simulink model "DOF2_Test2_arch"  (R2022b)
settings: Solver=VariableStepAuto  StartTime=0.0  StopTime=10.0  RelTol=1e-3
settings Model: Creator=shailesh suthar  LastModifiedBy=shailesh suthar
settings DebuggingCC: UnconnectedInputMsg=warning  UnconnectedOutputMsg=warning  UnconnectedLineMsg=warning
settings ModelReferenceCC: EnableRefExpFcnMdlSchedulingChecks=on
settings RTWCC: DLArmComputeVersion=19.05

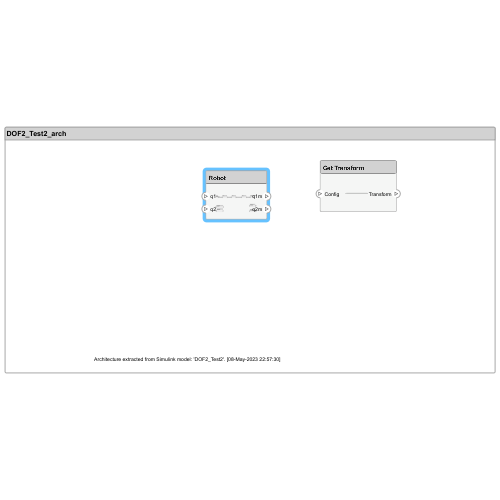
[thumbnail: Simulink's stored preview of the top-level diagram]
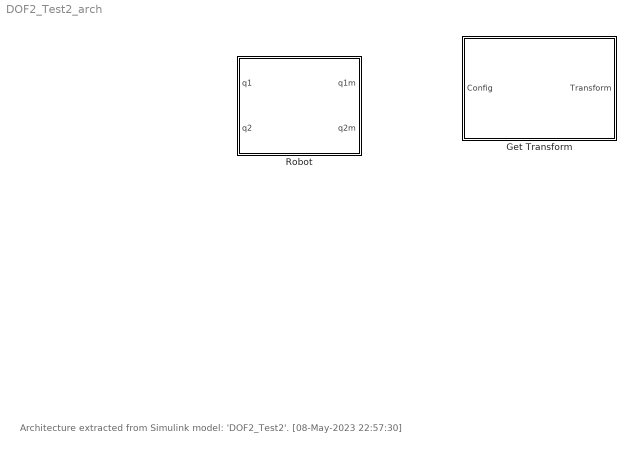
== system DOF2_Test2_arch ==
  note: Architecture extracted from Simulink model: 'DOF2_Test2'. [08-May-2023 22:57:30]
  Get Transform : Subsystem
      settings: PortSchema="{\"entries\":[{\"content\":{\"headerSize\":26,\"margin\":15,\"minimumSpacing\":25,\"sides\":[{\"content\":{\"connectorIds\":[\"In1\"]},\"type\":\"ConnectorPlacement.EquallySpacedRectSide\",\"uuid\":\"557e2789-5bde-45a7-9208-ef64bda35799\"},{\"content\":{\"connectorIds\":[\"Out1\"],\"side\":\"RIGHT\"},\"type\":\"ConnectorPlacement.EquallySpacedRectSide\",\"uuid\":\"adadcf43-a05c-4dbc-9e15-d3b2757a8feb\"},{\"content\":{\"connectorIds\":[],\"side\":\"TOP\"},\"type\":\"ConnectorPlacement.EquallySpacedRectSide\",\"uuid\":\"69984c12-afd6-46f7-91b1-af5b61a3164f\"}]},\"type\":\"ConnectorPlacement.EquallySpacedConnector\",\"uuid\":\"3da93d72-b13d-4c5c-bd73-b6426386ab06\"}],\"packageUris\":[\"http://schema.mathworks.com/mf0/Connector/R2020b\"],\"version\":\"1.0\"}"
  Robot : Subsystem
      settings: PortSchema="{\"entries\":[{\"content\":{\"headerSize\":26,\"margin\":15,\"minimumSpacing\":25,\"sides\":[{\"content\":{\"connectorIds\":[\"In1\",\"In2\"]},\"type\":\"ConnectorPlacement.EquallySpacedRectSide\",\"uuid\":\"557e2789-5bde-45a7-9208-ef64bda35799\"},{\"content\":{\"connectorIds\":[\"Out1\",\"Out2\"],\"side\":\"RIGHT\"},\"type\":\"ConnectorPlacement.EquallySpacedRectSide\",\"uuid\":\"adadcf43-a05c-4dbc-9e15-d3b2757a8feb\"},{\"content\":{\"connectorIds\":[],\"side\":\"TOP\"},\"type\":\"ConnectorPlacement.EquallySpacedRectSide\",\"uuid\":\"69984c12-afd6-46f7-91b1-af5b61a3164f\"}]},\"type\":\"ConnectorPlacement.EquallySpacedConnector\",\"uuid\":\"3da93d72-b13d-4c5c-bd73-b6426386ab06\"}],\"packageUris\":[\"http://schema.mathworks.com/mf0/Connector/R2020b\"],\"version\":\"1.0\"}"

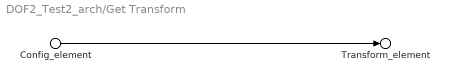
== system DOF2_Test2_arch/Get Transform ==
  Config_element : Inport  PortName=Config
  Transform_element : Outport  PortName=Transform
  wires:
  Config_element/1 -> Transform_element/1

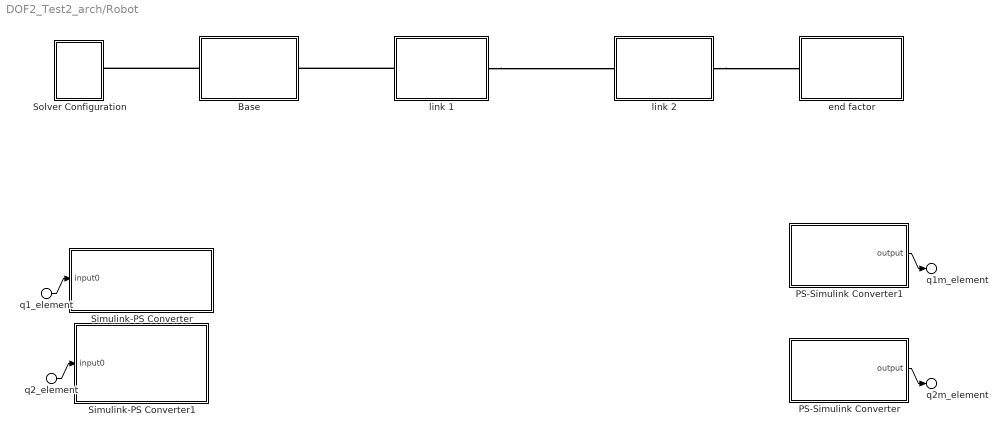
== system DOF2_Test2_arch/Robot ==
  q1_element : Inport  PortName=q1
  q2_element : Inport  Port=2  PortName=q2
  Base : Subsystem
      settings: PortSchema="{\"entries\":[{\"content\":{\"headerSize\":26,\"margin\":15,\"minimumSpacing\":25,\"sides\":[{\"content\":{\"connectorIds\":[\"LConn1\"]},\"type\":\"ConnectorPlacement.EquallySpacedRectSide\",\"uuid\":\"557e2789-5bde-45a7-9208-ef64bda35799\"},{\"content\":{\"connectorIds\":[\"RConn1\"],\"side\":\"RIGHT\"},\"type\":\"ConnectorPlacement.EquallySpacedRectSide\",\"uuid\":\"adadcf43-a05c-4dbc-9e15-d3b2757a8feb\"},{\"content\":{\"connectorIds\":[],\"side\":\"TOP\"},\"type\":\"ConnectorPlacement.EquallySpacedRectSide\",\"uuid\":\"69984c12-afd6-46f7-91b1-af5b61a3164f\"}]},\"type\":\"ConnectorPlacement.EquallySpacedConnector\",\"uuid\":\"3da93d72-b13d-4c5c-bd73-b6426386ab06\"}],\"packageUris\":[\"http://schema.mathworks.com/mf0/Connector/R2020b\"],\"version\":\"1.0\"}"
  PS-Simulink Converter : Subsystem  mask{Frequencies=[]}
      settings: PortSchema="{\"entries\":[{\"content\":{\"headerSize\":26,\"margin\":15,\"minimumSpacing\":25,\"sides\":[{\"content\":{\"connectorIds\":[\"LConn1\"]},\"type\":\"ConnectorPlacement.EquallySpacedRectSide\",\"uuid\":\"557e2789-5bde-45a7-9208-ef64bda35799\"},{\"content\":{\"connectorIds\":[\"Out1\"],\"side\":\"RIGHT\"},\"type\":\"ConnectorPlacement.EquallySpacedRectSide\",\"uuid\":\"adadcf43-a05c-4dbc-9e15-d3b2757a8feb\"},{\"content\":{\"connectorIds\":[],\"side\":\"TOP\"},\"type\":\"ConnectorPlacement.EquallySpacedRectSide\",\"uuid\":\"69984c12-afd6-46f7-91b1-af5b61a3164f\"}]},\"type\":\"ConnectorPlacement.EquallySpacedConnector\",\"uuid\":\"3da93d72-b13d-4c5c-bd73-b6426386ab06\"}],\"packageUris\":[\"http://schema.mathworks.com/mf0/Connector/R2020b\"],\"version\":\"1.0\"}"
  PS-Simulink Converter1 : Subsystem  mask{Frequencies=[]}
      settings: PortSchema="{\"entries\":[{\"content\":{\"headerSize\":26,\"margin\":15,\"minimumSpacing\":25,\"sides\":[{\"content\":{\"connectorIds\":[\"LConn1\"]},\"type\":\"ConnectorPlacement.EquallySpacedRectSide\",\"uuid\":\"557e2789-5bde-45a7-9208-ef64bda35799\"},{\"content\":{\"connectorIds\":[\"Out1\"],\"side\":\"RIGHT\"},\"type\":\"ConnectorPlacement.EquallySpacedRectSide\",\"uuid\":\"adadcf43-a05c-4dbc-9e15-d3b2757a8feb\"},{\"content\":{\"connectorIds\":[],\"side\":\"TOP\"},\"type\":\"ConnectorPlacement.EquallySpacedRectSide\",\"uuid\":\"69984c12-afd6-46f7-91b1-af5b61a3164f\"}]},\"type\":\"ConnectorPlacement.EquallySpacedConnector\",\"uuid\":\"3da93d72-b13d-4c5c-bd73-b6426386ab06\"}],\"packageUris\":[\"http://schema.mathworks.com/mf0/Connector/R2020b\"],\"version\":\"1.0\"}"
  Simulink-PS Converter : Subsystem  mask{Frequencies=[], NoiseParameters=[], InputFilterTimeConstant=[]}
      settings: PortSchema="{\"entries\":[{\"content\":{\"headerSize\":26,\"margin\":15,\"minimumSpacing\":25,\"sides\":[{\"content\":{\"connectorIds\":[\"In1\"]},\"type\":\"ConnectorPlacement.EquallySpacedRectSide\",\"uuid\":\"557e2789-5bde-45a7-9208-ef64bda35799\"},{\"content\":{\"connectorIds\":[\"RConn1\"],\"side\":\"RIGHT\"},\"type\":\"ConnectorPlacement.EquallySpacedRectSide\",\"uuid\":\"adadcf43-a05c-4dbc-9e15-d3b2757a8feb\"},{\"content\":{\"connectorIds\":[],\"side\":\"TOP\"},\"type\":\"ConnectorPlacement.EquallySpacedRectSide\",\"uuid\":\"69984c12-afd6-46f7-91b1-af5b61a3164f\"}]},\"type\":\"ConnectorPlacement.EquallySpacedConnector\",\"uuid\":\"3da93d72-b13d-4c5c-bd73-b6426386ab06\"}],\"packageUris\":[\"http://schema.mathworks.com/mf0/Connector/R2020b\"],\"version\":\"1.0\"}"
  Simulink-PS Converter1 : Subsystem  mask{Frequencies=[], NoiseParameters=[], InputFilterTimeConstant=[]}
      settings: PortSchema="{\"entries\":[{\"content\":{\"headerSize\":26,\"margin\":15,\"minimumSpacing\":25,\"sides\":[{\"content\":{\"connectorIds\":[\"In1\"]},\"type\":\"ConnectorPlacement.EquallySpacedRectSide\",\"uuid\":\"557e2789-5bde-45a7-9208-ef64bda35799\"},{\"content\":{\"connectorIds\":[\"RConn1\"],\"side\":\"RIGHT\"},\"type\":\"ConnectorPlacement.EquallySpacedRectSide\",\"uuid\":\"adadcf43-a05c-4dbc-9e15-d3b2757a8feb\"},{\"content\":{\"connectorIds\":[],\"side\":\"TOP\"},\"type\":\"ConnectorPlacement.EquallySpacedRectSide\",\"uuid\":\"69984c12-afd6-46f7-91b1-af5b61a3164f\"}]},\"type\":\"ConnectorPlacement.EquallySpacedConnector\",\"uuid\":\"3da93d72-b13d-4c5c-bd73-b6426386ab06\"}],\"packageUris\":[\"http://schema.mathworks.com/mf0/Connector/R2020b\"],\"version\":\"1.0\"}"
  Solver Configuration : Subsystem  mask{Tones=[], Harmonics=[], ResidualTolerance=[], ConsistencyAbsTol=[], ConsistencyRelTol=[], ConsistencyTolFactor=[], FunctionEvalNumThread=[], LocalSolverSampleTime=[], MaxNonlinIter=[], MaxModeIter=[], ImpulseIterations=[], LinearAlgebraNumThread=[], DelaysMemoryBudget=[], FilteringTimeConstant=[], PartitionMemoryBudget=[]}
      settings: PortSchema="{\"entries\":[{\"content\":{\"headerSize\":26,\"margin\":15,\"minimumSpacing\":25,\"sides\":[{\"content\":{\"connectorIds\":[]},\"type\":\"ConnectorPlacement.EquallySpacedRectSide\",\"uuid\":\"557e2789-5bde-45a7-9208-ef64bda35799\"},{\"content\":{\"connectorIds\":[\"RConn1\"],\"side\":\"RIGHT\"},\"type\":\"ConnectorPlacement.EquallySpacedRectSide\",\"uuid\":\"adadcf43-a05c-4dbc-9e15-d3b2757a8feb\"},{\"content\":{\"connectorIds\":[],\"side\":\"TOP\"},\"type\":\"ConnectorPlacement.EquallySpacedRectSide\",\"uuid\":\"69984c12-afd6-46f7-91b1-af5b61a3164f\"}]},\"type\":\"ConnectorPlacement.EquallySpacedConnector\",\"uuid\":\"3da93d72-b13d-4c5c-bd73-b6426386ab06\"}],\"packageUris\":[\"http://schema.mathworks.com/mf0/Connector/R2020b\"],\"version\":\"1.0\"}"
  end factor : Subsystem
      settings: PortSchema="{\"entries\":[{\"content\":{\"headerSize\":26,\"margin\":15,\"minimumSpacing\":25,\"sides\":[{\"content\":{\"connectorIds\":[\"LConn1\"]},\"type\":\"ConnectorPlacement.EquallySpacedRectSide\",\"uuid\":\"557e2789-5bde-45a7-9208-ef64bda35799\"},{\"content\":{\"connectorIds\":[],\"side\":\"RIGHT\"},\"type\":\"ConnectorPlacement.EquallySpacedRectSide\",\"uuid\":\"adadcf43-a05c-4dbc-9e15-d3b2757a8feb\"},{\"content\":{\"connectorIds\":[],\"side\":\"TOP\"},\"type\":\"ConnectorPlacement.EquallySpacedRectSide\",\"uuid\":\"69984c12-afd6-46f7-91b1-af5b61a3164f\"}]},\"type\":\"ConnectorPlacement.EquallySpacedConnector\",\"uuid\":\"3da93d72-b13d-4c5c-bd73-b6426386ab06\"}],\"packageUris\":[\"http://schema.mathworks.com/mf0/Connector/R2020b\"],\"version\":\"1.0\"}"
  link 1 : Subsystem
      settings: PortSchema="{\"entries\":[{\"content\":{\"headerSize\":26,\"margin\":15,\"minimumSpacing\":25,\"sides\":[{\"content\":{\"connectorIds\":[\"LConn1\"]},\"type\":\"ConnectorPlacement.EquallySpacedRectSide\",\"uuid\":\"557e2789-5bde-45a7-9208-ef64bda35799\"},{\"content\":{\"connectorIds\":[\"RConn1\"],\"side\":\"RIGHT\"},\"type\":\"ConnectorPlacement.EquallySpacedRectSide\",\"uuid\":\"adadcf43-a05c-4dbc-9e15-d3b2757a8feb\"},{\"content\":{\"connectorIds\":[],\"side\":\"TOP\"},\"type\":\"ConnectorPlacement.EquallySpacedRectSide\",\"uuid\":\"69984c12-afd6-46f7-91b1-af5b61a3164f\"}]},\"type\":\"ConnectorPlacement.EquallySpacedConnector\",\"uuid\":\"3da93d72-b13d-4c5c-bd73-b6426386ab06\"}],\"packageUris\":[\"http://schema.mathworks.com/mf0/Connector/R2020b\"],\"version\":\"1.0\"}"
  link 2 : Subsystem
      settings: PortSchema="{\"entries\":[{\"content\":{\"headerSize\":26,\"margin\":15,\"minimumSpacing\":25,\"sides\":[{\"content\":{\"connectorIds\":[\"LConn1\"]},\"type\":\"ConnectorPlacement.EquallySpacedRectSide\",\"uuid\":\"557e2789-5bde-45a7-9208-ef64bda35799\"},{\"content\":{\"connectorIds\":[\"RConn1\"],\"side\":\"RIGHT\"},\"type\":\"ConnectorPlacement.EquallySpacedRectSide\",\"uuid\":\"adadcf43-a05c-4dbc-9e15-d3b2757a8feb\"},{\"content\":{\"connectorIds\":[],\"side\":\"TOP\"},\"type\":\"ConnectorPlacement.EquallySpacedRectSide\",\"uuid\":\"69984c12-afd6-46f7-91b1-af5b61a3164f\"}]},\"type\":\"ConnectorPlacement.EquallySpacedConnector\",\"uuid\":\"3da93d72-b13d-4c5c-bd73-b6426386ab06\"}],\"packageUris\":[\"http://schema.mathworks.com/mf0/Connector/R2020b\"],\"version\":\"1.0\"}"
  q1m_element : Outport  PortName=q1m
  q2m_element : Outport  Port=2  PortName=q2m
  wires:
  q1_element/1 -> Simulink-PS Converter/1(input0)
  q2_element/1 -> Simulink-PS Converter1/1(input0)
  PS-Simulink Converter1/1(output) -> q1m_element/1
  PS-Simulink Converter/1(output) -> q2m_element/1
  connections:
  Base/LConn1 -- Solver Configuration/RConn1
  link 1/LConn1 -- Base/RConn1
  link 1/RConn1 -- link 2/LConn1
  link 2/RConn1 -- end factor/LConn1

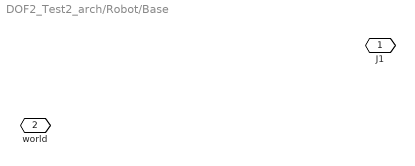
== system DOF2_Test2_arch/Robot/Base ==
  J1 : PMIOPort  Side=Right
  world : PMIOPort  Port=2  Side=Left

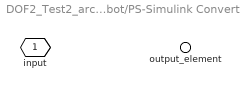
== system DOF2_Test2_arch/Robot/PS-Simulink Converter ==
  input : PMIOPort  Side=Left
  output_element : Outport  PortName=output

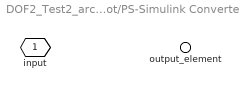
== system DOF2_Test2_arch/Robot/PS-Simulink Converter1 ==
  input : PMIOPort  Side=Left
  output_element : Outport  PortName=output

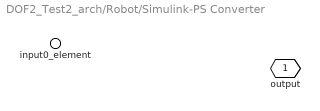
== system DOF2_Test2_arch/Robot/Simulink-PS Converter ==
  input0_element : Inport  PortName=input0
  output : PMIOPort  Side=Right

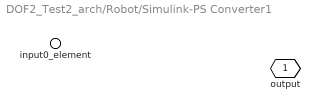
== system DOF2_Test2_arch/Robot/Simulink-PS Converter1 ==
  input0_element : Inport  PortName=input0
  output : PMIOPort  Side=Right

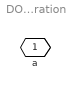
== system DOF2_Test2_arch/Robot/Solver Configuration ==
  a : PMIOPort  Side=Right

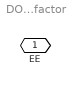
== system DOF2_Test2_arch/Robot/end factor ==
  EE : PMIOPort  Side=Left

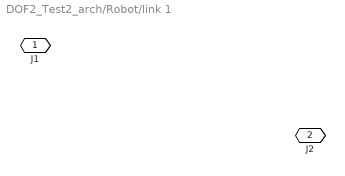
== system DOF2_Test2_arch/Robot/link 1 ==
  J1 : PMIOPort  Side=Left
  J2 : PMIOPort  Port=2  Side=Right

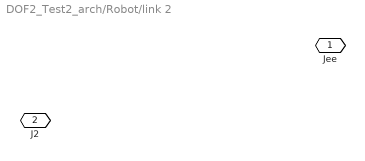
== system DOF2_Test2_arch/Robot/link 2 ==
  Jee : PMIOPort  Side=Right
  J2 : PMIOPort  Port=2  Side=Left
